simulink model "LyapunovDirectMethod"  (R2017a)
settings: Solver=VariableStepAuto  StartTime=0.0  StopTime=1000.0  RelTol=1e-3
undefined symbols (not defined in the file): alpha, C, M, Ro, theta, V
settings Model: Creator=HP  LastModifiedBy=HP

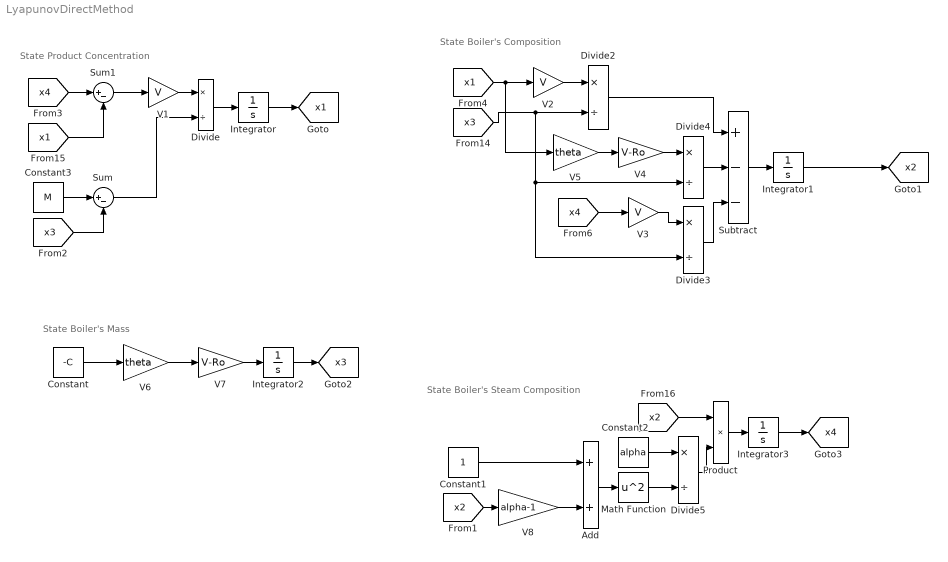
== system LyapunovDirectMethod ==
  note: State Boiler's Steam Composition
  note: State Boiler's Mass
  note: State Boiler's Composition
  note: State Product Concentration
  Add : Sum
  Constant : Constant  Value=-C
  Constant1 : Constant
  Constant2 : Constant  Value=alpha
  Constant3 : Constant  Value=M
  Divide{,2..5} (5 alike) : Product  Inputs=*/
  Integrator : Integrator  InitialCondition=0.85
  Integrator1 : Integrator  InitialCondition=0.113
  Integrator2 : Integrator  InitialCondition=130
  Integrator3 : Integrator  InitialCondition=0.8499
  Math Function : Math  Operator=square  SaturateOnIntegerOverflow=on
  Product : Product
  Subtract : Sum  Inputs=+--
  Sum : Sum  Inputs=|+-
  Sum1 : Sum  Inputs=|+-
  V1 : Gain  Gain=V
  V2 : Gain  Gain=V
  V3 : Gain  Gain=V
  V4 : Gain  Gain=V-Ro
  V5 : Gain  Gain=theta
  V6 : Gain  Gain=theta
  V7 : Gain  Gain=V-Ro
  V8 : Gain  Gain=alpha-1
  tag scope: x1=global, x2=global, x3=global, x4=global
  wires:
  Divide/1 -> Integrator/1
  [x1] -> V2/1, V5/1
  V2/1 -> Divide2/1
  [x4] -> V3/1
  V3/1 -> Divide3/1
  V5/1 -> V4/1
  V4/1 -> Divide4/1
  Divide2/1 -> Subtract/1
  Divide4/1 -> Subtract/2
  Divide3/1 -> Subtract/3
  Subtract/1 -> Integrator1/1
  Integrator1/1 -> [x2]
  V6/1 -> V7/1
  Integrator2/1 -> [x3]
  Constant/1 -> V6/1
  [x2] -> V8/1
  V8/1 -> Add/2
  Constant1/1 -> Add/1
  Add/1 -> Math Function/1
  Math Function/1 -> Divide5/2
  Constant2/1 -> Divide5/1
  Divide5/1 -> Product/2
  Product/1 -> Integrator3/1
  Integrator3/1 -> [x4]
  [x3] -> Sum/2
  Constant3/1 -> Sum/1
  V7/1 -> Integrator2/1
  V1/1 -> Divide/1
  Sum/1 -> Divide/2
  [x3] -> Divide3/2, Divide4/2, Divide2/2
  Sum1/1 -> V1/1
  [x4] -> Sum1/1
  [x1] -> Sum1/2
  Integrator/1 -> [x1]
  [x2] -> Product/1
